simulink model "pn_mod"  (Simulink 7.2)
settings: Solver=ode45  StartTime=0.0  StopTime=0.02  RelTol=1e-3
undefined symbols (not defined in the file or in its folder): Fs, get
libraries: dspsnks4 x2, commseqgen2 x1, commutil2 x1
settings Model: Creator=Administrator  LastModifiedBy=Administrator
settings OptimizationCC: InitFltsAndDblsToZero=on

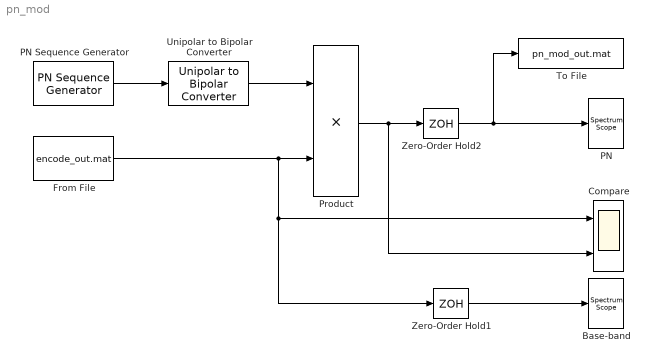
== system pn_mod ==
  Base-band : dspsnks4/Spectrum Scope  DialogController=dspdialog.SpectrumScope  DialogControllerArgs=DataTag0  SystemSampleTime=-1  ScopeProperties=on  Domain=Frequency  HorizSpan=1  UseBuffer=on  BufferSize=512  Overlap=256  inpFftLenInherit=off  FFTlength=128  numAvg=2  DisplayProperties=off  AxisGrid=on  Memory=off  FrameNumber=on  AxisLegend=off  AxisZoom=off  OpenScopeAtSimStart=on  OpenScopeImmediately=off  FigPos=get(0,'defaultfigureposition')  AxisProperties=off  XUnits=Hertz  XRange=[-Fs/2...Fs/2]  XDisplay=0  InheritXIncr=on  XIncr=1.0  XLabel=Samples  XLimit=Auto  YUnits=dB  XMax=1  XMin=0  YLabel=Magnitude-squared, dB  LineProperties=off  wintypeSpecScope=Hann  RsSpecScope=50  betaSpecScope=5  winsampSpecScope=Periodic
      settings: YMin=-29.4847114022419  YMax=22.1972278260597
  Compare : Scope  NumInputPorts=2
      settings: YMin=-5~-5  YMax=5~5
  From File : FromFile  FileName=encode_out.mat  SampleTime=1/1000
  PN : dspsnks4/Spectrum Scope  DialogController=dspdialog.SpectrumScope  DialogControllerArgs=DataTag1  SystemSampleTime=-1  ScopeProperties=on  Domain=Frequency  HorizSpan=1  UseBuffer=on  BufferSize=512  Overlap=256  inpFftLenInherit=off  FFTlength=128  numAvg=2  DisplayProperties=off  AxisGrid=on  Memory=off  FrameNumber=on  AxisLegend=off  AxisZoom=off  OpenScopeAtSimStart=on  OpenScopeImmediately=off  FigPos=get(0,'defaultfigureposition')  AxisProperties=off  XUnits=Hertz  XRange=[-Fs/2...Fs/2]  XDisplay=0  InheritXIncr=on  XIncr=1.0  XLabel=Samples  XLimit=Auto  YUnits=dB  XMax=1  XMin=0  YLabel=Magnitude-squared, dB  LineProperties=off  wintypeSpecScope=Hann  RsSpecScope=50  betaSpecScope=5  winsampSpecScope=Periodic
      settings: YMin=-57.0539933095568  YMax=14.6899176974794
  PN Sequence Generator : commseqgen2/PN Sequence Generator  poly=[1 0 0 0 1 1 1 0 1]  ini_sta=[0 0 0 0 0 0 0 1]  outBitMaskSource=Dialog parameter  shift=0  Ts=1/2.55e5  frameBased=off  sampPerFrame=1  reset=off  bitPackedOutputs=off  outDataType=double  numPackedBits=8  bitPackDataSigned=off  bitPackedOutDType=double
  Product : Product  OutDataType=sfix(16)  OutScaling=2^0  RndMeth=Zero
  To File : ToFile  Filename=pn_mod_out.mat
  Unipolar to Bipolar Converter : commutil2/Unipolar to Bipolar Converter  SystemSampleTime=-1  M=2  polarity=Positive  dataType=Same as input
  Zero-Order Hold1 : ZeroOrderHold  SampleTime=1/1e5
  Zero-Order Hold2 : ZeroOrderHold  SampleTime=1/2.55e6
  wires:
  PN Sequence Generator/1 -> Unipolar to Bipolar Converter/1
  Unipolar to Bipolar Converter/1 -> Product/1
  From File/1 -> Product/2, Zero-Order Hold1/1, Compare/1
  Product/1 -> Zero-Order Hold2/1, Compare/2
  Zero-Order Hold2/1 -> PN/1, To File/1
  Zero-Order Hold1/1 -> Base-band/1
